simulink model "SimlinkModel"  (R2022b)
settings: Solver=VariableStepAuto  StartTime=0.0  StopTime=5  RelTol=1e-3
undefined symbols (not defined in the file): eqmatrix, K, Ki
settings Model: Creator=Abdelateef  LastModifiedBy=عالم الكمبيوتر

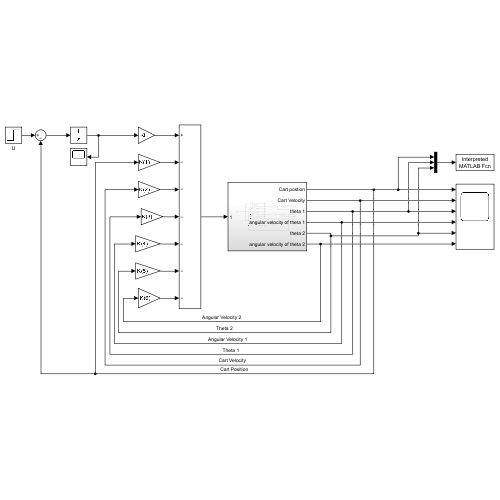
[thumbnail: Simulink's stored preview of the top-level diagram]
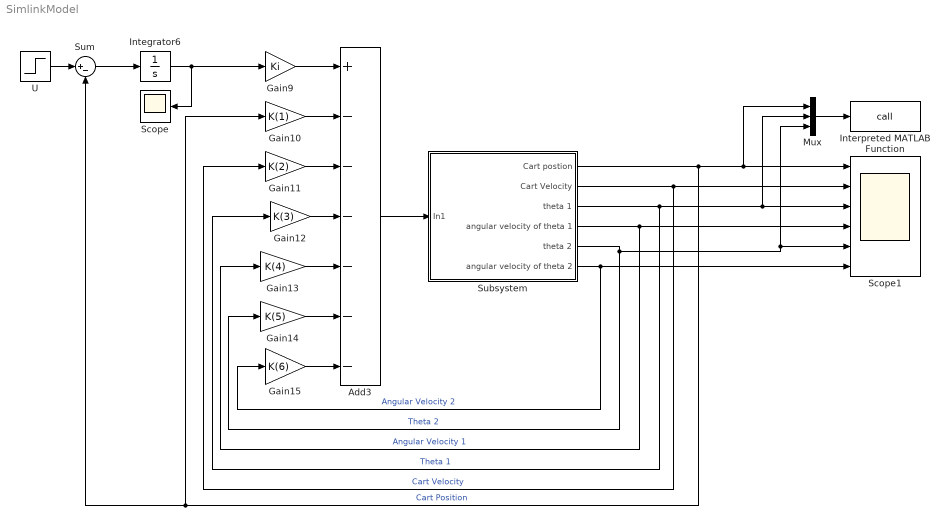
== system SimlinkModel ==
  Add3 : Sum  Inputs=+------
  Gain10 : Gain  Gain=K(1)
  Gain11 : Gain  Gain=K(2)
  Gain12 : Gain  Gain=K(3)
  Gain13 : Gain  Gain=K(4)
  Gain14 : Gain  Gain=K(5)
  Gain15 : Gain  Gain=K(6)
  Gain9 : Gain  Gain=Ki
  Integrator6 : Integrator
  Interpreted MATLAB Function : MATLABFcn  MATLABFcn=call  OutputDimensions=0
  Mux : Mux  Inputs=3
  Scope : Scope
  Scope1 : Scope  NumInputPorts=6
  Subsystem : Subsystem
  Sum : Sum  Inputs=|+-
  U : Step  SampleTime=0
  wires:
  U/1 -> Sum/1
  Integrator6/1 -> Scope/1, Gain9/1
  Gain9/1 -> Add3/1
  Gain10/1 -> Add3/2
  Gain11/1 -> Add3/3
  Gain12/1 -> Add3/4
  Gain13/1 -> Add3/5
  Gain14/1 -> Add3/6
  Gain15/1 -> Add3/7
  Sum/1 -> Integrator6/1
  Subsystem/1(Cart postion) -> Sum/2, Gain10/1, Mux/1, Scope1/1  "Cart Position"
  Add3/1 -> Subsystem/1(In1)
  Subsystem/2(Cart Velocity) -> Scope1/2, Gain11/1  "Cart Velocity"
  Subsystem/3(theta 1) -> Gain12/1, Mux/2, Scope1/3  "Theta 1"
  Subsystem/4(angular velocity of theta 1) -> Gain13/1, Scope1/4  "Angular Velocity 1"
  Subsystem/5(theta 2) -> Gain14/1, Mux/3, Scope1/5  "Theta 2"
  Subsystem/6(angular velocity of theta 2) -> Scope1/6, Gain15/1  "Angular Velocity 2"
  Mux/1 -> Interpreted MATLAB Function/1

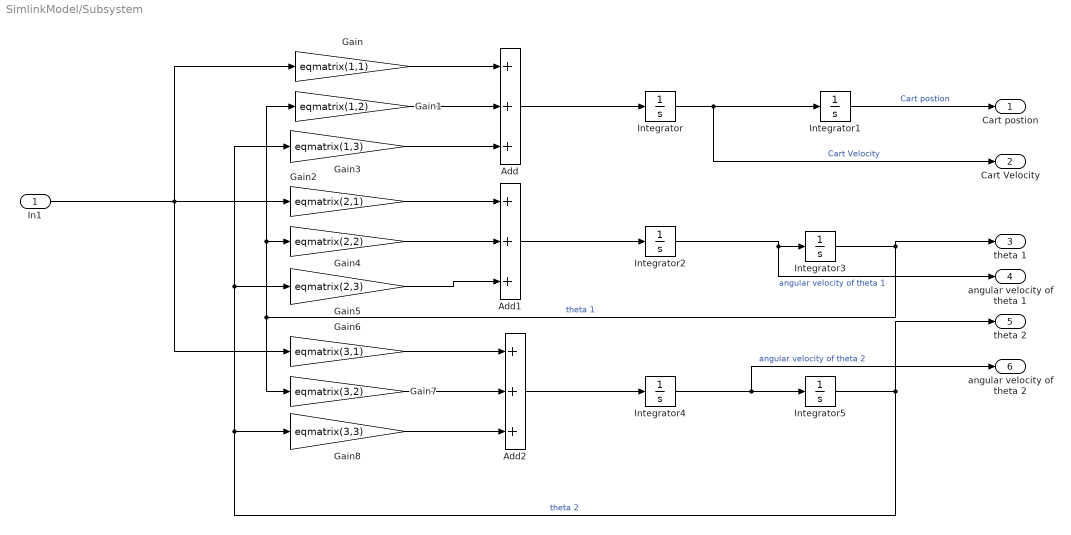
== system SimlinkModel/Subsystem ==
  In1 : Inport
  Add : Sum  Inputs=+++
  Add1 : Sum  Inputs=+++
  Add2 : Sum  Inputs=+++
  Gain : Gain  Gain=eqmatrix(1,1)
  Gain1 : Gain  Gain=eqmatrix(1,2)
  Gain2 : Gain  Gain=eqmatrix(2,1)
  Gain3 : Gain  Gain=eqmatrix(1,3)
  Gain4 : Gain  Gain=eqmatrix(2,2)
  Gain5 : Gain  Gain=eqmatrix(2,3)
  Gain6 : Gain  Gain=eqmatrix(3,1)
  Gain7 : Gain  Gain=eqmatrix(3,2)
  Gain8 : Gain  Gain=eqmatrix(3,3)
  Integrator{,1..5} (6 alike) : Integrator
  Cart postion : Outport
  Cart Velocity : Outport  Port=2
  theta 1 : Outport  Port=3
  angular velocity of theta 1 : Outport  Port=4
  theta 2 : Outport  Port=5
  angular velocity of theta 2 : Outport  Port=6
  wires:
  Gain2/1 -> Add1/1
  Gain4/1 -> Add1/2
  Integrator5/1 -> theta 2/1, Gain3/1, Gain5/1, Gain8/1  "theta 2"
  Integrator1/1 -> Cart postion/1  "Cart postion"
  Gain8/1 -> Add2/3
  Gain7/1 -> Add2/2
  Integrator4/1 -> angular velocity of theta 2/1, Integrator5/1  "angular velocity of theta 2"
  Integrator/1 -> Cart Velocity/1, Integrator1/1  "Cart Velocity"
  Integrator3/1 -> theta 1/1, Gain1/1, Gain4/1, Gain7/1  "theta 1"
  In1/1 -> Gain6/1, Gain2/1, Gain/1
  Gain1/1 -> Add/2
  Add/1 -> Integrator/1
  Gain3/1 -> Add/3
  Gain6/1 -> Add2/1
  Gain5/1 -> Add1/3
  Add2/1 -> Integrator4/1
  Integrator2/1 -> angular velocity of theta 1/1, Integrator3/1  "angular velocity of theta 1"
  Gain/1 -> Add/1
  Add1/1 -> Integrator2/1
